simulink model "matching"  (R2015a)
settings: Solver=ode45  StartTime=0.0  StopTime=10.0  RelTol=1e-3
InitFcn:
  | %% DSPBuilder Start
  | alt_dspbuilder_update_model(bdroot)
  | %% DSPBuilder End
libraries: allblocks_alteradspbuilder2 x186
(part 1 of 2)
settings Model: Creator=ASUS  LastModifiedBy=ASUS

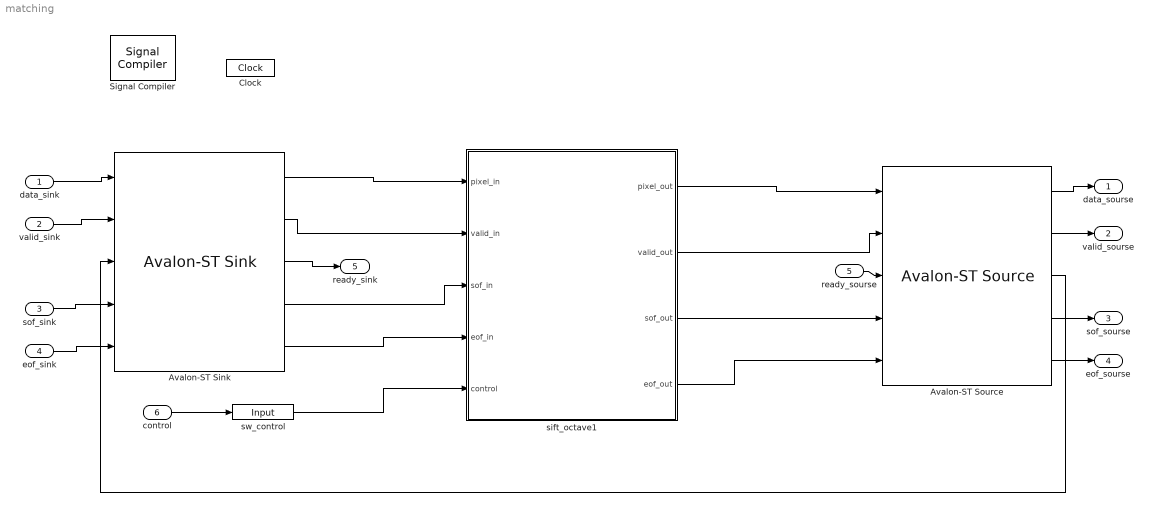
== system matching ==
  data_sink : Inport
  valid_sink : Inport  Port=2
  sof_sink : Inport  Port=3
  eof_sink : Inport  Port=4
  ready_sourse : Inport  Port=5
  control : Inport  Port=6
  Avalon-ST Sink : allblocks_alteradspbuilder2/Avalon-ST Sink  iofile=C:\Users\ASUS\Desktop\final_sift_fpga\tb_matching\matching_Avalon-ST+Sink_data.salt,C:\Users\ASUS\Desktop\final_sift_fpga\tb_matching\matching_Avalon-ST+Sink_valid.salt,C:\Users\ASUS\Desktop\final_sift_fpga\tb_matching\matching_Avalon-ST+Sink_ready.capture,C:\Users\ASUS\Desktop\final_sift_fpga\tb_matching\matching_Avalon-ST+Sink_startofpacket.salt,C:\Users\ASUS\Desktop\final_sift_fpga\tb_matching\matching_Avalon-ST+Sink_endofpacket.salt,  SpecifyClock=off  BusType=Unsigned Integer  bwl=24  bwr=0  symbolWidth=8  symbolsPerBeat=3  numOfChannels=0  numOfErrorDescriptors=0  endOfPacket=on  startOfPacket=on  empty=off  readyLatency=1  externalType=Inferred  PORTTYPE=Output
  Avalon-ST Source : allblocks_alteradspbuilder2/Avalon-ST Source  iofile=C:\Users\ASUS\Desktop\final_sift_fpga\tb_matching\matching_Avalon-ST+Source_data.capture,C:\Users\ASUS\Desktop\final_sift_fpga\tb_matching\matching_Avalon-ST+Source_valid.capture,C:\Users\ASUS\Desktop\final_sift_fpga\tb_matching\matching_Avalon-ST+Source_ready.salt,C:\Users\ASUS\Desktop\final_sift_fpga\tb_matching\matching_Avalon-ST+Source_startofpacket.capture,C:\Users\ASUS\Desktop\final_sift_fpga\tb_matching\matching_Avalon-ST+Source_endofpacket.capture,  SpecifyClock=off  BusType=Unsigned Integer  bwl=24  bwr=0  symbolWidth=8  symbolsPerBeat=3  numOfChannels=0  numOfErrorDescriptors=0  endOfPacket=on  startOfPacket=on  empty=off  readyLatency=1  externalType=Inferred  PORTTYPE=Input
  Clock : allblocks_alteradspbuilder2/Clock  ClockPeriod=10/1.5  ClockPeriodUnit=ns  SampleTime=1  ResetLatency=0  ResetRegisterCascadeDepth=0  SimulationStartCycle=5  PhaseOffset=0  Reset=aclr  ResetType=Active Low  Export=off
  Signal Compiler : allblocks_alteradspbuilder2/Signal Compiler  DeviceFamily=Cyclone IV GX  DeviceName=AUTO  DisableEarlyHDLGeneration=off  EnableSignalTap=off  SignalTapDepth=128  UseBoardBlock=off  StpUseDefaultClock=on  StpClock=Clock  ExportDir=C:\altera\16.0\quartus\dsp_builder  MAX10_ProgrammingMode=Internal Flash (SDM) Single Boot
  sift_octave1 : Subsystem
  sw_control : allblocks_alteradspbuilder2/Input  iofile=C:\Users\ASUS\Desktop\final_sift_fpga\tb_matching\matching_sw%5Fcontrol.salt  BusType=Unsigned Integer  bwl=18  bwr=0  SpecifyClock=off  PORTTYPE=Input  externalType=Inferred  allowFloatingPointOverride=on  logOutputs=off
  data_sourse : Outport
  valid_sourse : Outport  Port=2
  sof_sourse : Outport  Port=3
  eof_sourse : Outport  Port=4
  ready_sink : Outport  Port=5
  wires:
  sift_octave1/1(pixel_out) -> Avalon-ST Source/1
  Avalon-ST Sink/1 -> sift_octave1/1(pixel_in)
  Avalon-ST Sink/2 -> sift_octave1/2(valid_in)
  sift_octave1/2(valid_out) -> Avalon-ST Source/2
  sift_octave1/3(sof_out) -> Avalon-ST Source/4
  sift_octave1/4(eof_out) -> Avalon-ST Source/5
  Avalon-ST Sink/5 -> sift_octave1/4(eof_in)
  Avalon-ST Sink/4 -> sift_octave1/3(sof_in)
  Avalon-ST Source/3 -> Avalon-ST Sink/3
  Avalon-ST Source/1 -> data_sourse/1
  Avalon-ST Source/2 -> valid_sourse/1
  Avalon-ST Source/4 -> sof_sourse/1
  Avalon-ST Source/5 -> eof_sourse/1
  data_sink/1 -> Avalon-ST Sink/1
  valid_sink/1 -> Avalon-ST Sink/2
  sof_sink/1 -> Avalon-ST Sink/4
  eof_sink/1 -> Avalon-ST Sink/5
  ready_sourse/1 -> Avalon-ST Source/3
  Avalon-ST Sink/3 -> ready_sink/1
  control/1 -> sw_control/1
  sw_control/1 -> sift_octave1/5(control)

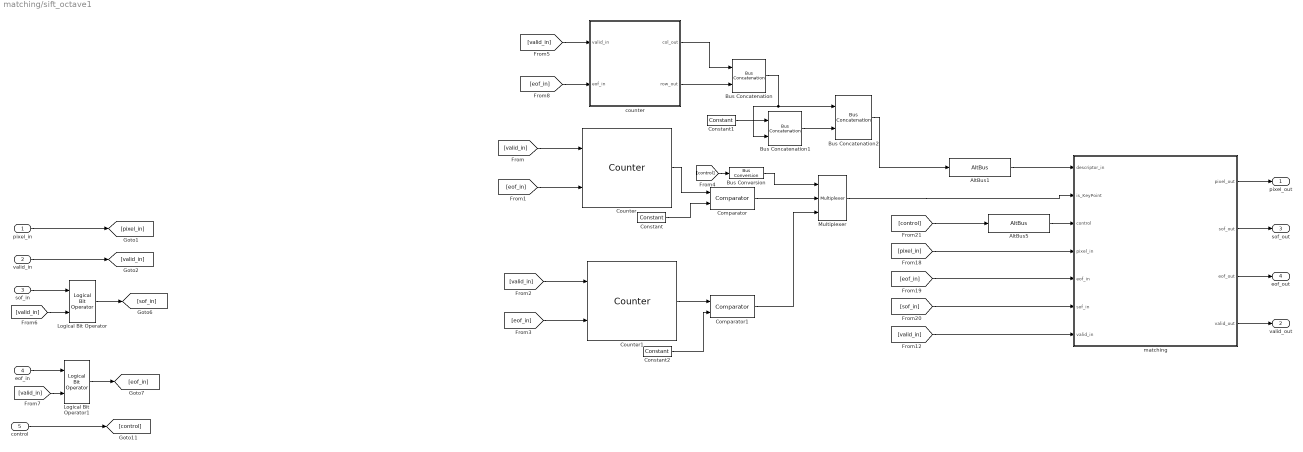
== system matching/sift_octave1 ==
  pixel_in : Inport
  valid_in : Inport  Port=2
  sof_in : Inport  Port=3
  eof_in : Inport  Port=4
  control : Inport  Port=5
  AltBus1 : allblocks_alteradspbuilder2/AltBus  BusType=Unsigned Integer  bwl=148  bwr=0  saturate=off  floatingPointInput=on  floatingPointOutput=on  logOutputs=off  logFile=C:\Users\ASUS\Desktop\final_sift_fpga\tb_matching\matching_sift%5Foctave1_AltBus1.fixedpointlog
  AltBus5 : allblocks_alteradspbuilder2/AltBus  BusType=Unsigned Integer  bwl=18  bwr=0  saturate=off  floatingPointInput=on  floatingPointOutput=on  logOutputs=off  logFile=C:\Users\ASUS\Desktop\final_sift_fpga\tb_matching\matching_sift%5Foctave1_AltBus5.fixedpointlog
  Bus Concatenation : allblocks_alteradspbuilder2/Bus Concatenation  isSigned=off  awidth=10  bwidth=10  pipeline_display=0
  Bus Concatenation1 : allblocks_alteradspbuilder2/Bus Concatenation  isSigned=off  awidth=108  bwidth=20  pipeline_display=0
  Bus Concatenation2 : allblocks_alteradspbuilder2/Bus Concatenation  isSigned=off  awidth=20  bwidth=128  pipeline_display=0
  Bus Conversion : allblocks_alteradspbuilder2/Bus Conversion  BusType=Unsigned Integer  ibwl=18  ibwr=1  bwl=1  bwr=1  bitToConnectToOutputLSB=17  round=off  saturate=off  pipeline_display=0
  Comparator : allblocks_alteradspbuilder2/Comparator  direction=a == b  pipeline_display=0  allowFloatingPointOverride=on  logOutputs=off  logFile=C:\Users\ASUS\Desktop\final_sift_fpga\tb_matching\matching_sift%5Foctave1_Comparator.fixedpointlog
  Comparator1 : allblocks_alteradspbuilder2/Comparator  direction=a == b  pipeline_display=0  allowFloatingPointOverride=on  logOutputs=off  logFile=C:\Users\ASUS\Desktop\final_sift_fpga\tb_matching\matching_sift%5Foctave1_Comparator1.fixedpointlog
  Constant : allblocks_alteradspbuilder2/Constant  mask_cst=5999  BusType=Unsigned Integer  bwl=20  bwr=0  roundMode=Truncate  satMode=Wrap  SpecifyClock=off  allowFloatingPointOverride=on  logOutputs=off  logFile=C:\Users\ASUS\Desktop\final_sift_fpga\tb_matching\matching_sift%5Foctave1_Constant.fixedpointlog
  Constant1 : allblocks_alteradspbuilder2/Constant  mask_cst=0  BusType=Unsigned Integer  bwl=108  bwr=0  roundMode=Truncate  satMode=Wrap  SpecifyClock=off  allowFloatingPointOverride=on  logOutputs=off  logFile=C:\Users\ASUS\Desktop\final_sift_fpga\tb_matching\matching_sift%5Foctave1_Constant1.fixedpointlog
  Constant2 : allblocks_alteradspbuilder2/Constant  mask_cst=4999  BusType=Unsigned Integer  bwl=20  bwr=0  roundMode=Truncate  satMode=Wrap  SpecifyClock=off  allowFloatingPointOverride=on  logOutputs=off  logFile=C:\Users\ASUS\Desktop\final_sift_fpga\tb_matching\matching_sift%5Foctave1_Constant2.fixedpointlog
  Counter : allblocks_alteradspbuilder2/Counter  BusType=Unsigned Integer  bwl=20  bwr=0  use_modulo=on  modulo=6000  SpecifyClock=off  direction=Increment  use_sload=off  use_sset=off  svalue=1  use_clk_ena=off  use_ena=on  use_sclr=on  pipeline_display=1
  Counter1 : allblocks_alteradspbuilder2/Counter  BusType=Unsigned Integer  bwl=20  bwr=0  use_modulo=on  modulo=5000  SpecifyClock=off  direction=Increment  use_sload=off  use_sset=off  svalue=1  use_clk_ena=off  use_ena=on  use_sclr=on  pipeline_display=1
  Logical Bit Operator : allblocks_alteradspbuilder2/Logical Bit Operator  LogicalOperator=AND  user_inputs=2  pipeline_display=0
  Logical Bit Operator1 : allblocks_alteradspbuilder2/Logical Bit Operator  LogicalOperator=AND  user_inputs=2  pipeline_display=0
  Multiplexer : allblocks_alteradspbuilder2/Multiplexer  numInputs=2  pipeline=0  oneHot=off  pipeline_display=0  use_ena=off  use_aclr=off  allowFloatingPointOverride=on  logOutputs=off  logFile=C:\Users\ASUS\Desktop\final_sift_fpga\tb_matching\matching_sift%5Foctave1_Multiplexer.fixedpointlog
  counter : Subsystem
  matching : Subsystem
  pixel_out : Outport
  valid_out : Outport  Port=2
  sof_out : Outport  Port=3
  eof_out : Outport  Port=4
  wires:
  control/1 -> [control]
  pixel_in/1 -> [pixel_in]
  valid_in/1 -> [valid_in]
  sof_in/1 -> Logical Bit Operator/1
  eof_in/1 -> Logical Bit Operator1/1
  AltBus1/1 -> matching/1(descriptor_in)
  [valid_in] -> matching/7(valid_in)
  [control] -> AltBus5/1
  [pixel_in] -> matching/4(pixel_in)
  [eof_in] -> matching/5(eof_in)
  [sof_in] -> matching/6(sof_in)
  AltBus5/1 -> matching/3(control)
  Comparator/1 -> Multiplexer/2
  [valid_in] -> counter/1(valid_in)
  [eof_in] -> counter/2(eof_in)
  counter/1(col_out) -> Bus Concatenation/1
  counter/2(row_out) -> Bus Concatenation/2
  Counter/1 -> Comparator/1
  [valid_in] -> Counter/1
  [eof_in] -> Counter/2
  Constant/1 -> Comparator/2
  Bus Concatenation/1 -> Bus Concatenation1/2, Bus Concatenation2/1
  Constant1/1 -> Bus Concatenation1/1
  Bus Concatenation1/1 -> Bus Concatenation2/2
  Bus Concatenation2/1 -> AltBus1/1
  Counter1/1 -> Comparator1/1
  [valid_in] -> Counter1/1
  [eof_in] -> Counter1/2
  Constant2/1 -> Comparator1/2
  Comparator1/1 -> Multiplexer/3
  Multiplexer/1 -> matching/2(is_KeyPoint)
  [control] -> Bus Conversion/1
  Bus Conversion/1 -> Multiplexer/1
  matching/1(pixel_out) -> pixel_out/1
  matching/2(sof_out) -> sof_out/1
  matching/3(eof_out) -> eof_out/1
  matching/4(valid_out) -> valid_out/1
  Logical Bit Operator/1 -> [sof_in]
  [valid_in] -> Logical Bit Operator/2
  Logical Bit Operator1/1 -> [eof_in]
  [valid_in] -> Logical Bit Operator1/2

== system matching/sift_octave1/counter ==
  valid_in : Inport
  eof_in : Inport  Port=2
  Comparator : allblocks_alteradspbuilder2/Comparator  direction=a == b  pipeline_display=0  allowFloatingPointOverride=on  logOutputs=off  logFile=C:\Users\ASUS\Desktop\PCIE_Display\custom_IP\tb_SIFT\SIFT_sift%5Foctave1_counter_Comparator.fixedpointlog
  Constant : allblocks_alteradspbuilder2/Constant  mask_cst=639  BusType=Unsigned Integer  bwl=10  bwr=0  roundMode=Truncate  satMode=Wrap  SpecifyClock=off  allowFloatingPointOverride=on  logOutputs=off  logFile=C:\Users\ASUS\Desktop\PCIE_Display\custom_IP\tb_SIFT\SIFT_sift%5Foctave1_counter_Constant.fixedpointlog
  Counter : allblocks_alteradspbuilder2/Counter  BusType=Unsigned Integer  bwl=10  bwr=0  use_modulo=on  modulo=640  SpecifyClock=off  direction=Increment  use_sload=off  use_sset=off  svalue=1  use_clk_ena=off  use_ena=on  use_sclr=on  pipeline_display=1
  Counter1 : allblocks_alteradspbuilder2/Counter  BusType=Unsigned Integer  bwl=10  bwr=0  use_modulo=on  modulo=480  SpecifyClock=off  direction=Increment  use_sload=off  use_sset=off  svalue=0  use_clk_ena=off  use_ena=on  use_sclr=on  pipeline_display=1
  Logical Bit Operator : allblocks_alteradspbuilder2/Logical Bit Operator  LogicalOperator=AND  user_inputs=2  pipeline_display=0
  col_out : Outport
  row_out : Outport  Port=2
  wires:
  [eof_in] -> Counter1/2
  Logical Bit Operator/1 -> Counter1/1
  [counter_col] -> Comparator/1
  eof_in/1 -> [eof_in]
  Constant/1 -> Comparator/2
  Comparator/1 -> Logical Bit Operator/2
  valid_in/1 -> [valid_in]
  Counter1/1 -> [counter_row]
  Counter/1 -> [counter_col]
  [valid_in] -> Logical Bit Operator/1, Counter/1
  [counter_row] -> row_out/1
  [counter_col] -> col_out/1
  [eof_in] -> Counter/2

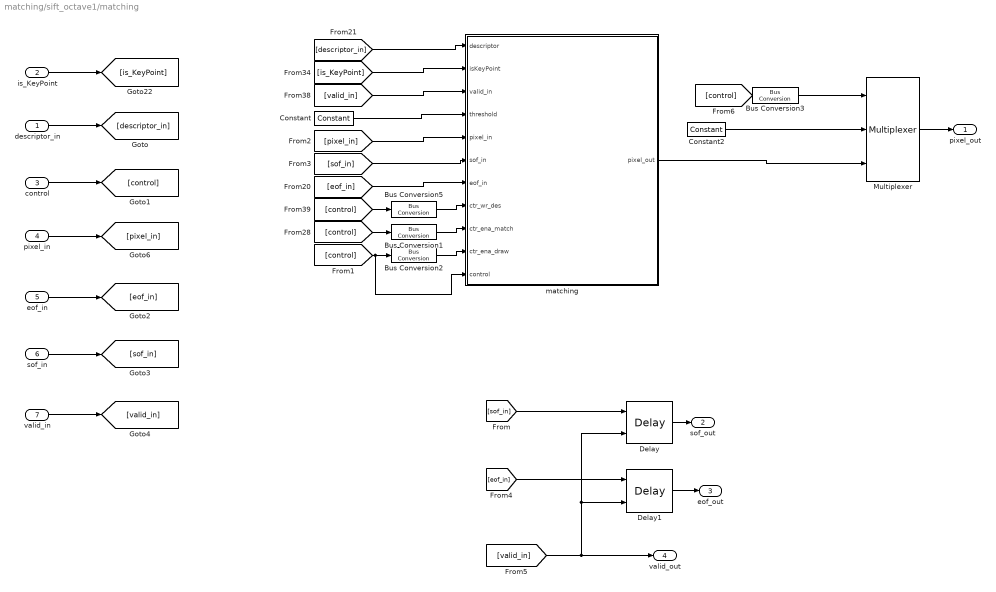
== system matching/sift_octave1/matching ==
  descriptor_in : Inport
  is_KeyPoint : Inport  Port=2
  control : Inport  Port=3
  pixel_in : Inport  Port=4
  eof_in : Inport  Port=5
  sof_in : Inport  Port=6
  valid_in : Inport  Port=7
  Bus Conversion1 : allblocks_alteradspbuilder2/Bus Conversion  BusType=Unsigned Integer  ibwl=18  ibwr=1  bwl=1  bwr=1  bitToConnectToOutputLSB=16  round=off  saturate=off  pipeline_display=0
  Bus Conversion2 : allblocks_alteradspbuilder2/Bus Conversion  BusType=Unsigned Integer  ibwl=18  ibwr=1  bwl=1  bwr=1  bitToConnectToOutputLSB=15  round=off  saturate=off  pipeline_display=0
  Bus Conversion3 : allblocks_alteradspbuilder2/Bus Conversion  BusType=Unsigned Integer  ibwl=18  ibwr=1  bwl=1  bwr=1  bitToConnectToOutputLSB=3  round=off  saturate=off  pipeline_display=0
  Bus Conversion5 : allblocks_alteradspbuilder2/Bus Conversion  BusType=Unsigned Integer  ibwl=18  ibwr=1  bwl=1  bwr=1  bitToConnectToOutputLSB=17  round=off  saturate=off  pipeline_display=0
  Constant : allblocks_alteradspbuilder2/Constant  mask_cst=1  BusType=Unsigned Integer  bwl=16  bwr=0  roundMode=Truncate  satMode=Wrap  SpecifyClock=off  allowFloatingPointOverride=on  logOutputs=off  logFile=C:\Users\ASUS\Desktop\final_sift_fpga\tb_matching\matching_sift%5Foctave1_matching_Constant.fixedpointlog
  Constant2 : allblocks_alteradspbuilder2/Constant  mask_cst=16711680  BusType=Unsigned Integer  bwl=24  bwr=0  roundMode=Truncate  satMode=Wrap  SpecifyClock=off  allowFloatingPointOverride=on  logOutputs=off  logFile=C:\Users\ASUS\Desktop\final_sift_fpga\tb_matching\matching_sift%5Foctave1_matching_Constant2.fixedpointlog
  Delay : allblocks_alteradspbuilder2/Delay  pipeline=4  pipeline_display=4  ClockPhase=1  use_ena=on  use_sclr=off  allowFloatingPointOverride=on  logOutputs=off  logFile=C:\Users\ASUS\Desktop\final_sift_fpga\tb_matching\matching_sift%5Foctave1_matching_Delay.fixedpointlog  use_init=off  reset_value=1
  Delay1 : allblocks_alteradspbuilder2/Delay  pipeline=4  pipeline_display=4  ClockPhase=1  use_ena=on  use_sclr=off  allowFloatingPointOverride=on  logOutputs=off  logFile=C:\Users\ASUS\Desktop\final_sift_fpga\tb_matching\matching_sift%5Foctave1_matching_Delay1.fixedpointlog  use_init=off  reset_value=1
  Multiplexer : allblocks_alteradspbuilder2/Multiplexer  numInputs=2  pipeline=0  oneHot=off  pipeline_display=0  use_ena=off  use_aclr=off  allowFloatingPointOverride=on  logOutputs=off  logFile=C:\Users\ASUS\Desktop\final_sift_fpga\tb_matching\matching_sift%5Foctave1_matching_Multiplexer.fixedpointlog
  matching : Subsystem
  pixel_out : Outport
  sof_out : Outport  Port=2
  eof_out : Outport  Port=3
  valid_out : Outport  Port=4
  wires:
  descriptor_in/1 -> [descriptor_in]
  control/1 -> [control]
  eof_in/1 -> [eof_in]
  sof_in/1 -> [sof_in]
  valid_in/1 -> [valid_in]
  pixel_in/1 -> [pixel_in]
  [descriptor_in] -> matching/1(descriptor)
  [is_KeyPoint] -> matching/2(isKeyPoint)
  [valid_in] -> matching/3(valid_in)
  Constant/1 -> matching/4(threshold)
  [eof_in] -> matching/7(eof_in)
  is_KeyPoint/1 -> [is_KeyPoint]
  [control] -> Bus Conversion5/1
  Bus Conversion5/1 -> matching/8(ctr_wr_des)
  [control] -> Bus Conversion1/1
  Bus Conversion1/1 -> matching/9(ctr_ena_match)
  [control] -> matching/11(control), Bus Conversion2/1
  Bus Conversion2/1 -> matching/10(ctr_ena_draw)
  [pixel_in] -> matching/5(pixel_in)
  [sof_in] -> matching/6(sof_in)
  [sof_in] -> Delay/1
  [eof_in] -> Delay1/1
  [valid_in] -> valid_out/1, Delay/2, Delay1/2
  Delay/1 -> sof_out/1
  Delay1/1 -> eof_out/1
  matching/1(pixel_out) -> Multiplexer/3
  Constant2/1 -> Multiplexer/2
  [control] -> Bus Conversion3/1
  Bus Conversion3/1 -> Multiplexer/1
  Multiplexer/1 -> pixel_out/1

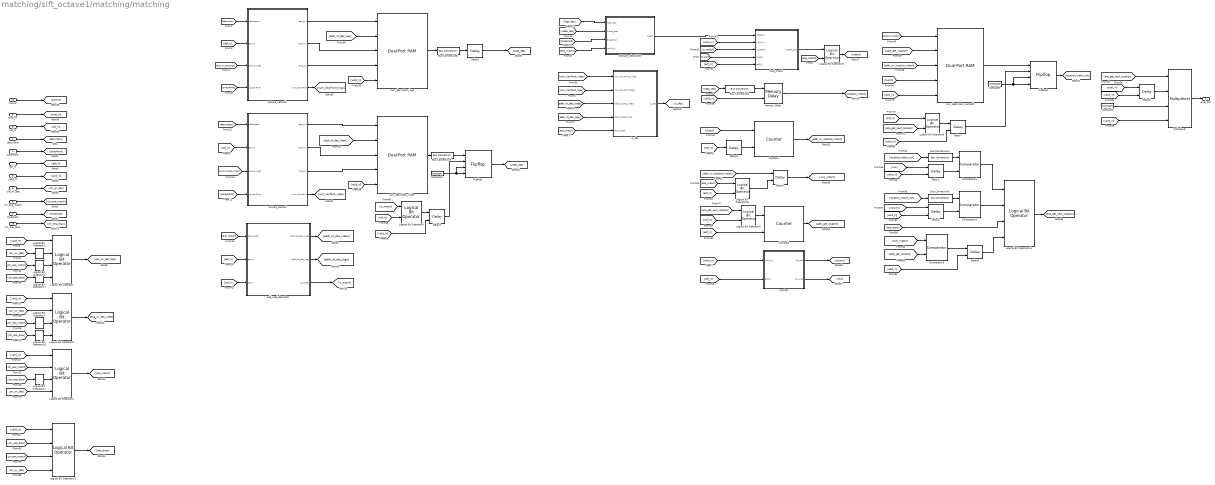
== system matching/sift_octave1/matching/matching ==
  descriptor : Inport
  isKeyPoint : Inport  Port=2
  valid_in : Inport  Port=3
  threshold : Inport  Port=4
  pixel_in : Inport  Port=5
  sof_in : Inport  Port=6
  eof_in : Inport  Port=7
  ctr_wr_des : Inport  Port=8
  ctr_ena_match : Inport  Port=9
  ctr_ena_draw : Inport  Port=10
  control : Inport  Port=11
  Bus Conversion3 : allblocks_alteradspbuilder2/Bus Conversion  BusType=Unsigned Integer  ibwl=148  ibwr=1  bwl=20  bwr=1  bitToConnectToOutputLSB=128  round=off  saturate=off  pipeline_display=0
  Bus Conversion4 : allblocks_alteradspbuilder2/Bus Conversion  BusType=Unsigned Integer  ibwl=20  ibwr=1  bwl=10  bwr=1  bitToConnectToOutputLSB=0  round=off  saturate=off  pipeline_display=0
  Bus Conversion5 : allblocks_alteradspbuilder2/Bus Conversion  BusType=Unsigned Integer  ibwl=20  ibwr=1  bwl=10  bwr=1  bitToConnectToOutputLSB=10  round=off  saturate=off  pipeline_display=0
  Bus Conversion6 : allblocks_alteradspbuilder2/Bus Conversion  BusType=Unsigned Integer  ibwl=148  ibwr=1  bwl=128  bwr=1  bitToConnectToOutputLSB=0  round=off  saturate=off  pipeline_display=0
  Bus Conversion7 : allblocks_alteradspbuilder2/Bus Conversion  BusType=Unsigned Integer  ibwl=148  ibwr=1  bwl=128  bwr=1  bitToConnectToOutputLSB=0  round=off  saturate=off  pipeline_display=0
  Comparator1 : allblocks_alteradspbuilder2/Comparator  direction=a == b  pipeline_display=0  allowFloatingPointOverride=on  logOutputs=off  logFile=C:\Users\ASUS\Desktop\final_sift_fpga\tb_matching\matching_sift%5Foctave1_matching_matching_Comparator1.fixedpointlog
  Comparator2 : allblocks_alteradspbuilder2/Comparator  direction=a == b  pipeline_display=0  allowFloatingPointOverride=on  logOutputs=off  logFile=C:\Users\ASUS\Desktop\final_sift_fpga\tb_matching\matching_sift%5Foctave1_matching_matching_Comparator2.fixedpointlog
  Comparator3 : allblocks_alteradspbuilder2/Comparator  direction=a >= b  pipeline_display=0  allowFloatingPointOverride=on  logOutputs=off  logFile=C:\Users\ASUS\Desktop\final_sift_fpga\tb_matching\matching_sift%5Foctave1_matching_matching_Comparator3.fixedpointlog
  Constant1 : allblocks_alteradspbuilder2/Constant  mask_cst=1  BusType=Single Bit  bwl=24  bwr=0  roundMode=Truncate  satMode=Wrap  SpecifyClock=off  allowFloatingPointOverride=on  logOutputs=off  logFile=C:\Users\ASUS\Desktop\final_sift_fpga\tb_matching\matching_sift%5Foctave1_matching_matching_Constant1.fixedpointlog
  Constant2 : allblocks_alteradspbuilder2/Constant  mask_cst=16711680  BusType=Unsigned Integer  bwl=24  bwr=0  roundMode=Truncate  satMode=Wrap  SpecifyClock=off  allowFloatingPointOverride=on  logOutputs=off  logFile=C:\Users\ASUS\Desktop\final_sift_fpga\tb_matching\matching_sift%5Foctave1_matching_matching_Constant2.fixedpointlog
  Constant3 : allblocks_alteradspbuilder2/Constant  mask_cst=1  BusType=Single Bit  bwl=24  bwr=0  roundMode=Truncate  satMode=Wrap  SpecifyClock=off  allowFloatingPointOverride=on  logOutputs=off  logFile=C:\Users\ASUS\Desktop\final_sift_fpga\tb_matching\matching_sift%5Foctave1_matching_matching_Constant3.fixedpointlog
  Counter1 : allblocks_alteradspbuilder2/Counter  BusType=Unsigned Integer  bwl=8  bwr=0  use_modulo=on  modulo=200  SpecifyClock=off  direction=Increment  use_sload=off  use_sset=off  svalue=1  use_clk_ena=off  use_ena=on  use_sclr=on  pipeline_display=1
  Counter2 : allblocks_alteradspbuilder2/Counter  BusType=Unsigned Integer  bwl=8  bwr=0  use_modulo=on  modulo=200  SpecifyClock=off  direction=Increment  use_sload=off  use_sset=off  svalue=1  use_clk_ena=off  use_ena=on  use_sclr=on  pipeline_display=1
  Delay1 : allblocks_alteradspbuilder2/Delay  pipeline=3  pipeline_display=3  ClockPhase=1  use_ena=on  use_sclr=off  allowFloatingPointOverride=on  logOutputs=off  logFile=C:\Users\ASUS\Desktop\final_sift_fpga\tb_matching\matching_sift%5Foctave1_matching_matching_Delay1.fixedpointlog  use_init=off  reset_value=1
  Delay2 : allblocks_alteradspbuilder2/Delay  pipeline=3  pipeline_display=3  ClockPhase=1  use_ena=on  use_sclr=off  allowFloatingPointOverride=on  logOutputs=off  logFile=C:\Users\ASUS\Desktop\final_sift_fpga\tb_matching\matching_sift%5Foctave1_matching_matching_Delay2.fixedpointlog  use_init=off  reset_value=1
  Delay3 : allblocks_alteradspbuilder2/Delay  pipeline=2  pipeline_display=2  ClockPhase=1  use_ena=on  use_sclr=off  allowFloatingPointOverride=on  logOutputs=off  logFile=C:\Users\ASUS\Desktop\final_sift_fpga\tb_matching\matching_sift%5Foctave1_matching_matching_Delay3.fixedpointlog  use_init=off  reset_value=1
  Delay4 : allblocks_alteradspbuilder2/Delay  pipeline=1  pipeline_display=1  ClockPhase=1  use_ena=on  use_sclr=off  allowFloatingPointOverride=on  logOutputs=off  logFile=C:\Users\ASUS\Desktop\final_sift_fpga\tb_matching\matching_sift%5Foctave1_matching_matching_Delay4.fixedpointlog  use_init=off  reset_value=1
  Delay5 : allblocks_alteradspbuilder2/Delay  pipeline=3  pipeline_display=3  ClockPhase=1  use_ena=on  use_sclr=off  allowFloatingPointOverride=on  logOutputs=off  logFile=C:\Users\ASUS\Desktop\final_sift_fpga\tb_matching\matching_sift%5Foctave1_matching_matching_Delay5.fixedpointlog  use_init=off  reset_value=1
  Delay6 : allblocks_alteradspbuilder2/Delay  pipeline=1  pipeline_display=1  ClockPhase=1  use_ena=off  use_sclr=off  allowFloatingPointOverride=on  logOutputs=off  logFile=C:\Users\ASUS\Desktop\final_sift_fpga\tb_matching\matching_sift%5Foctave1_matching_matching_Delay6.fixedpointlog  use_init=off  reset_value=1
  Delay7 : allblocks_alteradspbuilder2/Delay  pipeline=2  pipeline_display=2  ClockPhase=1  use_ena=on  use_sclr=off  allowFloatingPointOverride=on  logOutputs=off  logFile=C:\Users\ASUS\Desktop\final_sift_fpga\tb_matching\matching_sift%5Foctave1_matching_matching_Delay7.fixedpointlog  use_init=off  reset_value=1
  Delay8 : allblocks_alteradspbuilder2/Delay  pipeline=3  pipeline_display=3  ClockPhase=1  use_ena=on  use_sclr=off  allowFloatingPointOverride=on  logOutputs=off  logFile=C:\Users\ASUS\Desktop\final_sift_fpga\tb_matching\matching_sift%5Foctave1_matching_matching_Delay8.fixedpointlog  use_init=off  reset_value=1
  Delay9 : allblocks_alteradspbuilder2/Delay  pipeline=5  pipeline_display=5  ClockPhase=1  use_ena=off  use_sclr=off  allowFloatingPointOverride=on  logOutputs=off  logFile=C:\Users\ASUS\Desktop\final_sift_fpga\tb_matching\matching_sift%5Foctave1_matching_matching_Delay9.fixedpointlog  use_init=off  reset_value=1
  Flipflop1 : allblocks_alteradspbuilder2/Flipflop  mode=DFFE  BusType=Unsigned Integer  bwl=128  bwr=2  pipeline_display=1
  Flipflop2 : allblocks_alteradspbuilder2/Flipflop  mode=DFFE  BusType=Unsigned Integer  bwl=20  bwr=2  pipeline_display=1
  Logical Bit Operator{,2,5,14..15} (5 alike) : allblocks_alteradspbuilder2/Logical Bit Operator  LogicalOperator=AND  user_inputs=4  pipeline_display=0
  Logical Bit Operator{1,4,7,11,17..18} (6 alike) : allblocks_alteradspbuilder2/Logical Bit Operator  LogicalOperator=NOT  user_inputs=2  pipeline_display=0
  Logical Bit Operator16 : allblocks_alteradspbuilder2/Logical Bit Operator  LogicalOperator=AND  user_inputs=2  pipeline_display=0
  Logical Bit Operator3 : allblocks_alteradspbuilder2/Logical Bit Operator  LogicalOperator=OR  user_inputs=2  pipeline_display=0
  Logical Bit Operator6 : allblocks_alteradspbuilder2/Logical Bit Operator  LogicalOperator=OR  user_inputs=2  pipeline_display=0
  Logical Bit Operator8 : allblocks_alteradspbuilder2/Logical Bit Operator  LogicalOperator=OR  user_inputs=2  pipeline_display=0
  Logical Bit Operator9 : allblocks_alteradspbuilder2/Logical Bit Operator  LogicalOperator=AND  user_inputs=2  pipeline_display=0
  Memory Delay : allblocks_alteradspbuilder2/Memory Delay  BusType=Unsigned Integer  bwl=20  bwr=0  pipeline=211  pipeline_display=211  ram_type=AUTO  use_ena=on  use_sclr=off  allowFloatingPointOverride=on  logOutputs=off  logFile=C:\Users\ASUS\Desktop\final_sift_fpga\tb_matching\matching_sift%5Foctave1_matching_matching_Memory+Delay.fixedpointlog
  Multiplexer : allblocks_alteradspbuilder2/Multiplexer  numInputs=2  pipeline=1  oneHot=off  pipeline_display=1  use_ena=on  use_aclr=off  allowFloatingPointOverride=on  logOutputs=off  logFile=C:\Users\ASUS\Desktop\final_sift_fpga\tb_matching\matching_sift%5Foctave1_matching_matching_Multiplexer.fixedpointlog
  add_read_desciptor : Subsystem
  compare_descriptor : Subsystem
  counter : Subsystem
  final_match : Subsystem
  is_des : Subsystem
  picture_second : Subsystem
  picture_second1 : Subsystem
  ram_descriptor_logo : allblocks_alteradspbuilder2/Dual-Port RAM  numwords=200  BusType=Unsigned Integer  bwl=148  bwr=0  memory_type=AUTO  ram_type=DualRAM  dont_care=on  initialization=Blank  init_file=input.hex  init_array=[0:1:15]  register_outputs=on  use_ena=on  ClockPhase=1  allowFloatingPointOverride=on  logOutputs=off  logFile=C:\Users\ASUS\Desktop\final_sift_fpga\tb_matching\matching_sift%5Foctave1_matching_matching_ram%5Fdescriptor%5Flogo.fixedpointlog  pipeline_display=2
  ram_descriptor_second1 : allblocks_alteradspbuilder2/Dual-Port RAM  numwords=200  BusType=Unsigned Integer  bwl=20  bwr=0  memory_type=AUTO  ram_type=DualRAM  dont_care=on  initialization=Blank  init_file=input.hex  init_array=[0:1:15]  register_outputs=on  use_ena=on  ClockPhase=1  allowFloatingPointOverride=on  logOutputs=off  logFile=C:\Users\ASUS\Desktop\final_sift_fpga\tb_matching\matching_sift%5Foctave1_matching_matching_ram%5Fdescriptor%5Fsecond1.fixedpointlog  pipeline_display=2
  ram_descriptor_video : allblocks_alteradspbuilder2/Dual-Port RAM  numwords=1536  BusType=Unsigned Integer  bwl=148  bwr=0  memory_type=AUTO  ram_type=DualRAM  dont_care=on  initialization=Blank  init_file=input.hex  init_array=[0:1:15]  register_outputs=on  use_ena=on  ClockPhase=1  allowFloatingPointOverride=on  logOutputs=off  logFile=C:\Users\ASUS\Desktop\final_sift_fpga\tb_matching\matching_sift%5Foctave1_matching_matching_ram%5Fdescriptor%5Fvideo.fixedpointlog  pipeline_display=2
  pixel_out : Outport
  wires:
  descriptor/1 -> [descriptor]
  ctr_wr_des/1 -> [ctr_wr_des]
  eof_in/1 -> [eof_in]
  isKeyPoint/1 -> [isKeyPoint]
  valid_in/1 -> [valid_in]
  threshold/1 -> [threshold]
  Logical Bit Operator/1 -> [ena_wr_des_logo]
  [ctr_wr_des] -> Logical Bit Operator1/1
  [valid_in] -> Logical Bit Operator/1
  Logical Bit Operator1/1 -> Logical Bit Operator/2
  [ctr_ena_match] -> Logical Bit Operator4/1
  Logical Bit Operator4/1 -> Logical Bit Operator/3
  ctr_ena_match/1 -> [ctr_ena_match]
  Logical Bit Operator5/1 -> [ena_wr_des_video]
  [valid_in] -> Logical Bit Operator5/1
  [ctr_wr_des] -> Logical Bit Operator5/2
  [ctr_ena_match] -> Logical Bit Operator7/1
  Logical Bit Operator7/1 -> Logical Bit Operator5/3
  Logical Bit Operator2/1 -> [ena_match]
  [valid_in] -> Logical Bit Operator2/1
  [ctr_ena_match] -> Logical Bit Operator2/2
  ctr_ena_draw/1 -> [ctr_ena_draw]
  [ctr_ena_draw] -> Logical Bit Operator11/1
  Logical Bit Operator11/1 -> Logical Bit Operator2/3
  Logical Bit Operator15/1 -> [ena_draw]
  [valid_in] -> Logical Bit Operator15/1
  [ctr_ena_draw] -> Logical Bit Operator15/2
  pixel_in/1 -> [pixel_in]
  sof_in/1 -> [sof_in]
  [ctr_ena_draw] -> Logical Bit Operator17/1
  [ctr_ena_draw] -> Logical Bit Operator18/1
  Logical Bit Operator17/1 -> Logical Bit Operator/4
  Logical Bit Operator18/1 -> Logical Bit Operator5/4
  control/1 -> [control]
  [ctr_wr_des] -> Logical Bit Operator2/4
  [ctr_ena_match] -> Logical Bit Operator15/3
  [ctr_wr_des] -> Logical Bit Operator15/4
  [eof_in] -> picture_second/2(eof_in)
  ram_descriptor_video/1 -> Bus Conversion7/1
  [addr_rd_des_video] -> ram_descriptor_video/2
  picture_second/1(des_out) -> ram_descriptor_video/1
  picture_second/2(addr_wr) -> ram_descriptor_video/3
  [descriptor] -> picture_second/1(descriptor)
  [ena_wr_des_video] -> picture_second/3(ena_wr_des)
  [isKeyPoint] -> picture_second/4(is_KeyPoint)
  [ena_match] -> add_read_desciptor/1(ena_match)
  add_read_desciptor/1(addr_rd_des_video) -> [addr_rd_des_video]
  picture_second/3(ena_wr) -> ram_descriptor_video/4
  picture_second/4(num_KeyPoint) -> [num_KeyPoint_video]
  [eof_in] -> add_read_desciptor/2(eof_in)
  add_read_desciptor/3(is_match) -> [is_match]
  [sof_in] -> add_read_desciptor/3(sof_in)
  [descriptor] -> picture_second1/1(descriptor)
  [ena_wr_des_logo] -> picture_second1/3(ena_wr_des)
  [eof_in] -> picture_second1/2(eof_in)
  [isKeyPoint] -> picture_second1/4(is_KeyPoint)
  Multiplexer/1 -> pixel_out/1
  ram_descriptor_logo/1 -> Bus Conversion6/1
  [addr_rd_des_logo] -> ram_descriptor_logo/2
  picture_second1/1(des_out) -> ram_descriptor_logo/1
  picture_second1/2(addr_wr) -> ram_descriptor_logo/3
  picture_second1/3(ena_wr) -> ram_descriptor_logo/4
  picture_second1/4(num_KeyPoint) -> [num_KeyPoint_logo]
  add_read_desciptor/2(addr_rd_des_logo) -> [addr_rd_des_logo]
  [valid_in] -> ram_descriptor_logo/5
  [valid_in] -> ram_descriptor_video/5
  Flipflop1/1 -> [video_des]
  [is_match] -> Logical Bit Operator6/1
  [sof_in] -> Logical Bit Operator6/2
  Logical Bit Operator6/1 -> Delay3/1
  [valid_in] -> Delay3/2
  Delay3/1 -> Flipflop1/2
  Constant1/1 -> Flipflop1/3, Flipflop1/4
  Delay6/1 -> [logo_des]
  Bus Conversion6/1 -> Delay6/1
  Bus Conversion7/1 -> Flipflop1/1
  final_match/1(match_out) -> Logical Bit Operator9/1
  [pixel_in] -> Delay5/1
  [valid_in] -> Delay5/2
  Delay5/1 -> Multiplexer/2
  [valid_in] -> Multiplexer/4
  Constant2/1 -> Multiplexer/3
  [threshold] -> compare_descriptor/3(threshold)
  [ena_match] -> compare_descriptor/4(valid_in)
  [logo_des] -> compare_descriptor/1(logo_des)
  [video_des] -> compare_descriptor/2(video_des)
  compare_descriptor/1(match) -> final_match/1(match_in)
  [valid_in] -> final_match/2("valid_in ")
  [is_match] -> final_match/3(is_match)
  [is_des] -> final_match/4(is_des)
  [eof_in] -> final_match/5(eof_in)
  [num_KeyPoint_video] -> is_des/1(num_KeyPoint_video)
  [num_KeyPoint_logo] -> is_des/2(num_KeyPoint_logo)
  [addr_rd_des_video] -> is_des/3(addr_rd_des_video)
  [addr_rd_des_logo] -> is_des/4(addr_rd_des_logo)
  [ena_match] -> is_des/5(ena_match)
  is_des/1(is_des) -> [is_des]
  Bus Conversion3/1 -> Memory Delay/1
  [valid_in] -> Memory Delay/2
  [video_des] -> Bus Conversion3/1
  Counter1/1 -> [addr_wr_location_match]
  [eof_in] -> Delay9/1
  Counter2/1 -> [addr_get_location]
  [ena_get_next_location] -> Logical Bit Operator3/1
  [eof_in] -> Counter2/2
  [valid_in] -> counter/1(valid_in)
  [eof_in] -> counter/2(eof_in)
  counter/1(col_out) -> [column]
  counter/2(row_out) -> [row]
  [ena_match] -> Logical Bit Operator16/1
  [addr_wr_location_match] -> Delay4/1
  [eof_in] -> Logical Bit Operator16/2
  Logical Bit Operator16/1 -> Delay4/2
  Delay4/1 -> [num_match]
  Delay9/1 -> Counter1/2
  Logical Bit Operator3/1 -> Counter2/1
  [sof_in] -> Logical Bit Operator3/2
  Memory Delay/1 -> [location_match]
  [match] -> Counter1/1
  [ena_get_next_location] -> Multiplexer/1
  [location_match] -> ram_descriptor_second1/1
  [match] -> ram_descriptor_second1/4
  [addr_wr_location_match] -> ram_descriptor_second1/3
  ram_descriptor_second1/1 -> Flipflop2/1
  [addr_get_location] -> ram_descriptor_second1/2
  [location_match_out] -> Bus Conversion4/1
  Bus Conversion4/1 -> Comparator1/1
  [row] -> Delay1/1
  [location_match_out] -> Bus Conversion5/1
  Bus Conversion5/1 -> Comparator2/1
  Comparator2/1 -> Logical Bit Operator14/2
  Comparator1/1 -> Logical Bit Operator14/1
  [ena_draw] -> Logical Bit Operator14/3
  Logical Bit Operator14/1 -> [ena_get_next_location]
  Delay1/1 -> Comparator1/2
  [valid_in] -> Delay1/2
  [column] -> Delay2/1
  Delay2/1 -> Comparator2/2
  [valid_in] -> Delay2/2
  [num_match] -> Comparator3/1
  [addr_get_location] -> Comparator3/2
  Comparator3/1 -> Delay8/1
  [valid_in] -> ram_descriptor_second1/5
  Flipflop2/1 -> [location_match_out]
  [ena_get_next_location] -> Logical Bit Operator8/2
  [sof_in] -> Logical Bit Operator8/1
  Logical Bit Operator8/1 -> Delay7/1
  [valid_in] -> Delay7/2
  Delay7/1 -> Flipflop2/2
  Constant3/1 -> Flipflop2/3, Flipflop2/4
  Delay8/1 -> Logical Bit Operator14/4
  [valid_in] -> Delay8/2
  Logical Bit Operator9/1 -> [match]
  [ena_match] -> Logical Bit Operator9/2

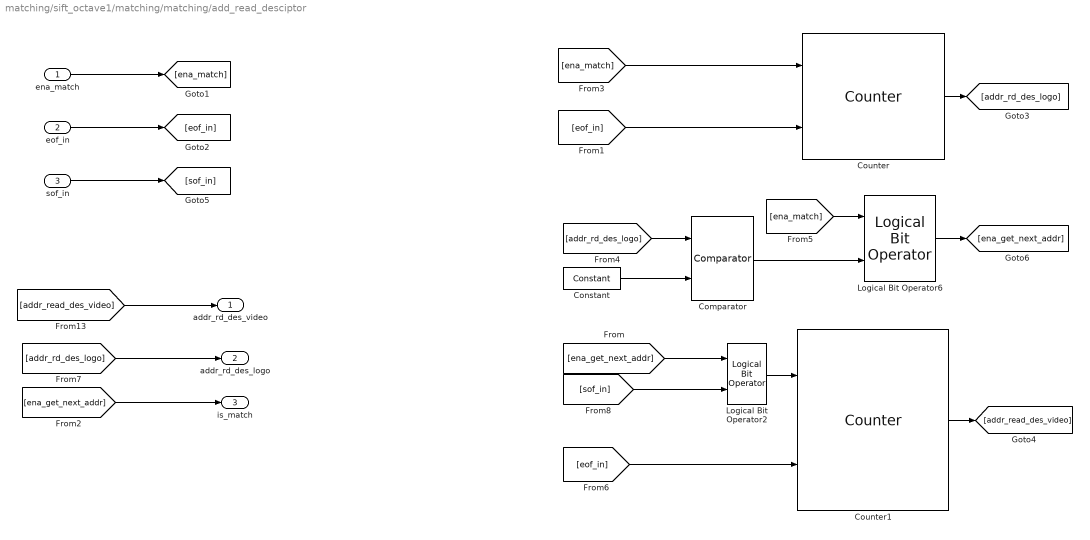
== system matching/sift_octave1/matching/matching/add_read_desciptor ==
  ena_match : Inport
  eof_in : Inport  Port=2
  sof_in : Inport  Port=3
  Comparator : allblocks_alteradspbuilder2/Comparator  direction=a == b  pipeline_display=0  allowFloatingPointOverride=on  logOutputs=off  logFile=C:\Users\ASUS\Desktop\PCIE_Display\custom_IP\tb_SIFT\SIFT_sift%5Foctave1_matching_matching_add%5Fread%5Fdesciptor_Comparator.fixedpointlog
  Constant : allblocks_alteradspbuilder2/Constant  mask_cst=199  BusType=Unsigned Integer  bwl=10  bwr=0  roundMode=Truncate  satMode=Wrap  SpecifyClock=off  allowFloatingPointOverride=on  logOutputs=off  logFile=C:\Users\ASUS\Desktop\PCIE_Display\custom_IP\tb_SIFT\SIFT_sift%5Foctave1_matching_matching_add%5Fread%5Fdesciptor_Constant.fixedpointlog
  Counter : allblocks_alteradspbuilder2/Counter  BusType=Unsigned Integer  bwl=8  bwr=0  use_modulo=on  modulo=200  SpecifyClock=off  direction=Increment  use_sload=off  use_sset=off  svalue=1  use_clk_ena=off  use_ena=on  use_sclr=on  pipeline_display=1
  Counter1 : allblocks_alteradspbuilder2/Counter  BusType=Unsigned Integer  bwl=11  bwr=0  use_modulo=on  modulo=1536  SpecifyClock=off  direction=Increment  use_sload=off  use_sset=off  svalue=0  use_clk_ena=off  use_ena=on  use_sclr=on  pipeline_display=1
  Logical Bit Operator2 : allblocks_alteradspbuilder2/Logical Bit Operator  LogicalOperator=OR  user_inputs=2  pipeline_display=0
  Logical Bit Operator6 : allblocks_alteradspbuilder2/Logical Bit Operator  LogicalOperator=AND  user_inputs=2  pipeline_display=0
  addr_rd_des_video : Outport
  addr_rd_des_logo : Outport  Port=2
  is_match : Outport  Port=3
  wires:
  [addr_rd_des_logo] -> Comparator/1
  ena_match/1 -> [ena_match]
  Constant/1 -> Comparator/2
  Counter1/1 -> [addr_read_des_video]
  Counter/1 -> [addr_rd_des_logo]
  [addr_read_des_video] -> addr_rd_des_video/1
  Comparator/1 -> Logical Bit Operator6/2
  [ena_match] -> Counter/1
  Logical Bit Operator6/1 -> [ena_get_next_addr]
  eof_in/1 -> [eof_in]
  [eof_in] -> Counter/2
  [ena_match] -> Logical Bit Operator6/1
  [ena_get_next_addr] -> is_match/1
  [eof_in] -> Counter1/2
  [ena_get_next_addr] -> Logical Bit Operator2/1
  sof_in/1 -> [sof_in]
  Logical Bit Operator2/1 -> Counter1/1
  [sof_in] -> Logical Bit Operator2/2
  [addr_rd_des_logo] -> addr_rd_des_logo/1

== system matching/sift_octave1/matching/matching/compare_descriptor ==
  logo_des : Inport
  video_des : Inport  Port=2
  threshold : Inport  Port=3
  valid_in : Inport  Port=4
  AltBus2 : allblocks_alteradspbuilder2/AltBus  BusType=Unsigned Integer  bwl=16  bwr=0  saturate=off  floatingPointInput=on  floatingPointOutput=on  logOutputs=off  logFile=C:\Users\ASUS\Desktop\final_sift_fpga\tb_matching\matching_sift%5Foctave1_matching_matching_compare%5Fdescriptor_AltBus2.fixedpointlog
  AltBus3 : allblocks_alteradspbuilder2/AltBus  BusType=Unsigned Integer  bwl=16  bwr=0  saturate=off  floatingPointInput=on  floatingPointOutput=on  logOutputs=off  logFile=C:\Users\ASUS\Desktop\final_sift_fpga\tb_matching\matching_sift%5Foctave1_matching_matching_compare%5Fdescriptor_AltBus3.fixedpointlog
  Delay : allblocks_alteradspbuilder2/Delay  pipeline=4  pipeline_display=4  ClockPhase=1  use_ena=on  use_sclr=off  allowFloatingPointOverride=on  logOutputs=off  logFile=C:\Users\ASUS\Desktop\final_sift_fpga\tb_matching\matching_sift%5Foctave1_matching_matching_compare%5Fdescriptor_Delay.fixedpointlog  use_init=off  reset_value=1
  Delay1 : allblocks_alteradspbuilder2/Delay  pipeline=1  pipeline_display=1  ClockPhase=1  use_ena=on  use_sclr=off  allowFloatingPointOverride=on  logOutputs=off  logFile=C:\Users\ASUS\Desktop\final_sift_fpga\tb_matching\matching_sift%5Foctave1_matching_matching_compare%5Fdescriptor_Delay1.fixedpointlog  use_init=off  reset_value=1
  compare : Subsystem
  get_distance : Subsystem
  match : Outport
  wires:
  [clken] -> get_distance/3(clken)
  video_des/1 -> get_distance/2(hist_in2)
  logo_des/1 -> get_distance/1(hist_in1)
  get_distance/1(distance_out) -> [distance]
  threshold/1 -> [threshold]
  Delay/1 -> AltBus3/1
  [threshold] -> AltBus2/1
  [match] -> match/1
  compare/1(match) -> Delay1/1
  AltBus2/1 -> compare/1(threshold)
  AltBus3/1 -> compare/2(distance)
  valid_in/1 -> [clken]
  [distance] -> Delay/1
  [clken] -> Delay/2
  Delay1/1 -> [match]
  [clken] -> Delay1/2

== system matching/sift_octave1/matching/matching/counter ==
  valid_in : Inport
  eof_in : Inport  Port=2
  Comparator : allblocks_alteradspbuilder2/Comparator  direction=a == b  pipeline_display=0  allowFloatingPointOverride=on  logOutputs=off  logFile=C:\Users\ASUS\Desktop\PCIE_Display\custom_IP\tb_SIFT\SIFT_sift%5Foctave1_matching_matching_counter_Comparator.fixedpointlog
  Constant : allblocks_alteradspbuilder2/Constant  mask_cst=639  BusType=Unsigned Integer  bwl=10  bwr=0  roundMode=Truncate  satMode=Wrap  SpecifyClock=off  allowFloatingPointOverride=on  logOutputs=off  logFile=C:\Users\ASUS\Desktop\PCIE_Display\custom_IP\tb_SIFT\SIFT_sift%5Foctave1_matching_matching_counter_Constant.fixedpointlog
  Counter : allblocks_alteradspbuilder2/Counter  BusType=Unsigned Integer  bwl=10  bwr=0  use_modulo=on  modulo=640  SpecifyClock=off  direction=Increment  use_sload=off  use_sset=off  svalue=1  use_clk_ena=off  use_ena=on  use_sclr=on  pipeline_display=1
  Counter1 : allblocks_alteradspbuilder2/Counter  BusType=Unsigned Integer  bwl=10  bwr=0  use_modulo=on  modulo=480  SpecifyClock=off  direction=Increment  use_sload=off  use_sset=off  svalue=0  use_clk_ena=off  use_ena=on  use_sclr=on  pipeline_display=1
  Logical Bit Operator : allblocks_alteradspbuilder2/Logical Bit Operator  LogicalOperator=AND  user_inputs=2  pipeline_display=0
  col_out : Outport
  row_out : Outport  Port=2
  wires:
  [eof_in] -> Counter1/2
  Logical Bit Operator/1 -> Counter1/1
  [counter_col] -> Comparator/1
  eof_in/1 -> [eof_in]
  Constant/1 -> Comparator/2
  Comparator/1 -> Logical Bit Operator/2
  valid_in/1 -> [valid_in]
  Counter1/1 -> [counter_row]
  Counter/1 -> [counter_col]
  [valid_in] -> Logical Bit Operator/1, Counter/1
  [counter_row] -> row_out/1
  [counter_col] -> col_out/1
  [eof_in] -> Counter/2

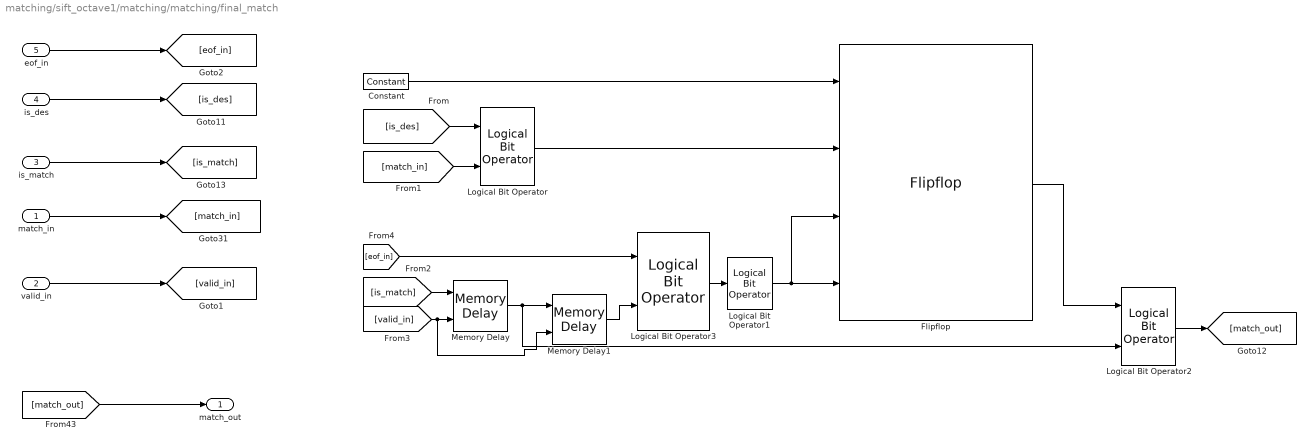
== system matching/sift_octave1/matching/matching/final_match ==
  match_in : Inport
  "valid_in " : Inport  Port=2
  is_match : Inport  Port=3
  is_des : Inport  Port=4
  eof_in : Inport  Port=5
  Constant : allblocks_alteradspbuilder2/Constant  mask_cst=1  BusType=Single Bit  bwl=8  bwr=0  roundMode=Truncate  satMode=Wrap  SpecifyClock=off  allowFloatingPointOverride=on  logOutputs=off  logFile=C:\Users\ASUS\Desktop\PCIE_Display\custom_IP\tb_SIFT\SIFT_sift%5Foctave1_matching_matching_final%5Fmatch_Constant.fixedpointlog
  Flipflop : allblocks_alteradspbuilder2/Flipflop  mode=DFFE  BusType=Single Bit  bwl=2  bwr=2  pipeline_display=1
  Logical Bit Operator : allblocks_alteradspbuilder2/Logical Bit Operator  LogicalOperator=AND  user_inputs=2  pipeline_display=0
  Logical Bit Operator1 : allblocks_alteradspbuilder2/Logical Bit Operator  LogicalOperator=NOT  user_inputs=2  pipeline_display=0
  Logical Bit Operator2 : allblocks_alteradspbuilder2/Logical Bit Operator  LogicalOperator=AND  user_inputs=2  pipeline_display=0
  Logical Bit Operator3 : allblocks_alteradspbuilder2/Logical Bit Operator  LogicalOperator=OR  user_inputs=2  pipeline_display=0
  Memory Delay : allblocks_alteradspbuilder2/Memory Delay  BusType=Unsigned Integer  bwl=1  bwr=0  pipeline=12  pipeline_display=12  ram_type=AUTO  use_ena=on  use_sclr=off  allowFloatingPointOverride=on  logOutputs=off  logFile=C:\Users\ASUS\Desktop\PCIE_Display\custom_IP\tb_SIFT\SIFT_sift%5Foctave1_matching_matching_final%5Fmatch_Memory+Delay.fixedpointlog
  Memory Delay1 : allblocks_alteradspbuilder2/Memory Delay  BusType=Unsigned Integer  bwl=1  bwr=0  pipeline=1  pipeline_display=1  ram_type=AUTO  use_ena=on  use_sclr=off  allowFloatingPointOverride=on  logOutputs=off  logFile=C:\Users\ASUS\Desktop\PCIE_Display\custom_IP\tb_SIFT\SIFT_sift%5Foctave1_matching_matching_final%5Fmatch_Memory+Delay1.fixedpointlog
  match_out : Outport
  wires:
  "valid_in "/1 -> [valid_in]
  match_in/1 -> [match_in]
  [match_out] -> match_out/1
  is_match/1 -> [is_match]
  is_des/1 -> [is_des]
  Flipflop/1 -> Logical Bit Operator2/1
  Constant/1 -> Flipflop/1
  [is_des] -> Logical Bit Operator/1
  [match_in] -> Logical Bit Operator/2
  Logical Bit Operator/1 -> Flipflop/2
  [is_match] -> Memory Delay/1
  [valid_in] -> Memory Delay1/2, Memory Delay/2
  Logical Bit Operator1/1 -> Flipflop/3, Flipflop/4
  Memory Delay/1 -> Memory Delay1/1, Logical Bit Operator2/2
  Logical Bit Operator2/1 -> [match_out]
  eof_in/1 -> [eof_in]
  Logical Bit Operator3/1 -> Logical Bit Operator1/1
  [eof_in] -> Logical Bit Operator3/1
  Memory Delay1/1 -> Logical Bit Operator3/2

== system matching/sift_octave1/matching/matching/is_des ==
  num_KeyPoint_video : Inport
  num_KeyPoint_logo : Inport  Port=2
  addr_rd_des_video : Inport  Port=3
  addr_rd_des_logo : Inport  Port=4
  ena_match : Inport  Port=5
  Comparator : allblocks_alteradspbuilder2/Comparator  direction=a >= b  pipeline_display=0  allowFloatingPointOverride=on  logOutputs=off  logFile=C:\Users\ASUS\Desktop\PCIE_Display\custom_IP\tb_SIFT\SIFT_sift%5Foctave1_matching_matching_is%5Fdes_Comparator.fixedpointlog
  Comparator6 : allblocks_alteradspbuilder2/Comparator  direction=a >= b  pipeline_display=0  allowFloatingPointOverride=on  logOutputs=off  logFile=C:\Users\ASUS\Desktop\PCIE_Display\custom_IP\tb_SIFT\SIFT_sift%5Foctave1_matching_matching_is%5Fdes_Comparator6.fixedpointlog
  Logical Bit Operator9 : allblocks_alteradspbuilder2/Logical Bit Operator  LogicalOperator=AND  user_inputs=2  pipeline_display=0
  Memory Delay1 : allblocks_alteradspbuilder2/Memory Delay  BusType=Unsigned Integer  bwl=1  bwr=0  pipeline=13  pipeline_display=13  ram_type=AUTO  use_ena=on  use_sclr=off  allowFloatingPointOverride=on  logOutputs=off  logFile=C:\Users\ASUS\Desktop\PCIE_Display\custom_IP\tb_SIFT\SIFT_sift%5Foctave1_matching_matching_is%5Fdes_Memory+Delay1.fixedpointlog
  Memory Delay2 : allblocks_alteradspbuilder2/Memory Delay  BusType=Unsigned Integer  bwl=1  bwr=0  pipeline=13  pipeline_display=13  ram_type=AUTO  use_ena=on  use_sclr=off  allowFloatingPointOverride=on  logOutputs=off  logFile=C:\Users\ASUS\Desktop\PCIE_Display\custom_IP\tb_SIFT\SIFT_sift%5Foctave1_matching_matching_is%5Fdes_Memory+Delay2.fixedpointlog
  is_des : Outport
  wires:
  [num_KeyPoint_video] -> Comparator/1
  Comparator/1 -> Memory Delay2/1
  [addr_rd_des_video] -> Comparator/2
  [ena_match] -> Memory Delay2/2
  [num_KeyPoint_logo] -> Comparator6/1
  Comparator6/1 -> Memory Delay1/1
  [addr_rd_des_logo] -> Comparator6/2
  Memory Delay2/1 -> Logical Bit Operator9/1
  Memory Delay1/1 -> Logical Bit Operator9/2
  Logical Bit Operator9/1 -> is_des/1
  [ena_match] -> Memory Delay1/2
  num_KeyPoint_video/1 -> [num_KeyPoint_video]
  num_KeyPoint_logo/1 -> [num_KeyPoint_logo]
  addr_rd_des_video/1 -> [addr_rd_des_video]
  addr_rd_des_logo/1 -> [addr_rd_des_logo]
  ena_match/1 -> [ena_match]

== system matching/sift_octave1/matching/matching/picture_second ==
  descriptor : Inport
  eof_in : Inport  Port=2
  ena_wr_des : Inport  Port=3
  is_KeyPoint : Inport  Port=4
  Constant1 : allblocks_alteradspbuilder2/Constant  mask_cst=1  BusType=Single Bit  bwl=24  bwr=0  roundMode=Truncate  satMode=Wrap  SpecifyClock=off  allowFloatingPointOverride=on  logOutputs=off  logFile=C:\Users\ASUS\Desktop\PCIE_Display\custom_IP\tb_SIFT\SIFT_sift%5Foctave1_matching_matching_picture%5Fsecond_Constant1.fixedpointlog
  Counter : allblocks_alteradspbuilder2/Counter  BusType=Unsigned Integer  bwl=11  bwr=0  use_modulo=on  modulo=1536  SpecifyClock=off  direction=Increment  use_sload=off  use_sset=off  svalue=1  use_clk_ena=off  use_ena=on  use_sclr=on  pipeline_display=1
  Delay1 : allblocks_alteradspbuilder2/Delay  pipeline=1  pipeline_display=1  ClockPhase=1  use_ena=on  use_sclr=off  allowFloatingPointOverride=on  logOutputs=off  logFile=C:\Users\ASUS\Desktop\PCIE_Display\custom_IP\tb_SIFT\SIFT_sift%5Foctave1_matching_matching_picture%5Fsecond_Delay1.fixedpointlog  use_init=off  reset_value=1
  Delay2 : allblocks_alteradspbuilder2/Delay  pipeline=5  pipeline_display=5  ClockPhase=1  use_ena=on  use_sclr=off  allowFloatingPointOverride=on  logOutputs=off  logFile=C:\Users\ASUS\Desktop\PCIE_Display\custom_IP\tb_SIFT\SIFT_sift%5Foctave1_matching_matching_picture%5Fsecond_Delay2.fixedpointlog  use_init=off  reset_value=1
  Delay3 : allblocks_alteradspbuilder2/Delay  pipeline=1  pipeline_display=1  ClockPhase=1  use_ena=on  use_sclr=off  allowFloatingPointOverride=on  logOutputs=off  logFile=C:\Users\ASUS\Desktop\PCIE_Display\custom_IP\tb_SIFT\SIFT_sift%5Foctave1_matching_matching_picture%5Fsecond_Delay3.fixedpointlog  use_init=off  reset_value=1
  Delay4 : allblocks_alteradspbuilder2/Delay  pipeline=1  pipeline_display=1  ClockPhase=1  use_ena=on  use_sclr=off  allowFloatingPointOverride=on  logOutputs=off  logFile=C:\Users\ASUS\Desktop\PCIE_Display\custom_IP\tb_SIFT\SIFT_sift%5Foctave1_matching_matching_picture%5Fsecond_Delay4.fixedpointlog  use_init=off  reset_value=1
  Flipflop : allblocks_alteradspbuilder2/Flipflop  mode=DFFE  BusType=Unsigned Integer  bwl=148  bwr=2  pipeline_display=1
  Logical Bit Operator1 : allblocks_alteradspbuilder2/Logical Bit Operator  LogicalOperator=AND  user_inputs=2  pipeline_display=0
  Logical Bit Operator4 : allblocks_alteradspbuilder2/Logical Bit Operator  LogicalOperator=AND  user_inputs=2  pipeline_display=0
  des_out : Outport
  addr_wr : Outport  Port=2
  ena_wr : Outport  Port=3
  num_KeyPoint : Outport  Port=4
  wires:
  descriptor/1 -> Flipflop/1
  Logical Bit Operator4/1 -> Flipflop/2, Delay3/1, Counter/1
  is_KeyPoint/1 -> Logical Bit Operator4/1
  Delay1/1 -> num_KeyPoint/1
  Counter/1 -> Delay4/1, Delay1/1
  Delay2/1 -> Counter/2
  eof_in/1 -> Logical Bit Operator1/1, Delay2/1
  ena_wr_des/1 -> Logical Bit Operator1/2, Delay2/2, Logical Bit Operator4/2, Delay4/2, Delay3/2
  Logical Bit Operator1/1 -> Delay1/2
  Flipflop/1 -> des_out/1
  Constant1/1 -> Flipflop/3, Flipflop/4
  Delay3/1 -> ena_wr/1
  Delay4/1 -> addr_wr/1

== system matching/sift_octave1/matching/matching/picture_second1 ==
  descriptor : Inport
  eof_in : Inport  Port=2
  ena_wr_des : Inport  Port=3
  is_KeyPoint : Inport  Port=4
  Constant1 : allblocks_alteradspbuilder2/Constant  mask_cst=1  BusType=Single Bit  bwl=24  bwr=0  roundMode=Truncate  satMode=Wrap  SpecifyClock=off  allowFloatingPointOverride=on  logOutputs=off  logFile=C:\Users\ASUS\Desktop\PCIE_Display\custom_IP\tb_SIFT\SIFT_sift%5Foctave1_matching_matching_picture%5Fsecond1_Constant1.fixedpointlog
  Counter : allblocks_alteradspbuilder2/Counter  BusType=Unsigned Integer  bwl=8  bwr=0  use_modulo=on  modulo=200  SpecifyClock=off  direction=Increment  use_sload=off  use_sset=off  svalue=1  use_clk_ena=off  use_ena=on  use_sclr=on  pipeline_display=1
  Delay1 : allblocks_alteradspbuilder2/Delay  pipeline=1  pipeline_display=1  ClockPhase=1  use_ena=on  use_sclr=off  allowFloatingPointOverride=on  logOutputs=off  logFile=C:\Users\ASUS\Desktop\PCIE_Display\custom_IP\tb_SIFT\SIFT_sift%5Foctave1_matching_matching_picture%5Fsecond1_Delay1.fixedpointlog  use_init=off  reset_value=1
  Delay2 : allblocks_alteradspbuilder2/Delay  pipeline=5  pipeline_display=5  ClockPhase=1  use_ena=on  use_sclr=off  allowFloatingPointOverride=on  logOutputs=off  logFile=C:\Users\ASUS\Desktop\PCIE_Display\custom_IP\tb_SIFT\SIFT_sift%5Foctave1_matching_matching_picture%5Fsecond1_Delay2.fixedpointlog  use_init=off  reset_value=1
  Delay3 : allblocks_alteradspbuilder2/Delay  pipeline=1  pipeline_display=1  ClockPhase=1  use_ena=on  use_sclr=off  allowFloatingPointOverride=on  logOutputs=off  logFile=C:\Users\ASUS\Desktop\PCIE_Display\custom_IP\tb_SIFT\SIFT_sift%5Foctave1_matching_matching_picture%5Fsecond1_Delay3.fixedpointlog  use_init=off  reset_value=1
  Delay4 : allblocks_alteradspbuilder2/Delay  pipeline=1  pipeline_display=1  ClockPhase=1  use_ena=on  use_sclr=off  allowFloatingPointOverride=on  logOutputs=off  logFile=C:\Users\ASUS\Desktop\PCIE_Display\custom_IP\tb_SIFT\SIFT_sift%5Foctave1_matching_matching_picture%5Fsecond1_Delay4.fixedpointlog  use_init=off  reset_value=1
  Flipflop : allblocks_alteradspbuilder2/Flipflop  mode=DFFE  BusType=Unsigned Integer  bwl=148  bwr=2  pipeline_display=1
  Logical Bit Operator1 : allblocks_alteradspbuilder2/Logical Bit Operator  LogicalOperator=AND  user_inputs=2  pipeline_display=0
  Logical Bit Operator4 : allblocks_alteradspbuilder2/Logical Bit Operator  LogicalOperator=AND  user_inputs=2  pipeline_display=0
  des_out : Outport
  addr_wr : Outport  Port=2
  ena_wr : Outport  Port=3
  num_KeyPoint : Outport  Port=4
  wires:
  descriptor/1 -> Flipflop/1
  Logical Bit Operator4/1 -> Flipflop/2, Delay3/1, Counter/1
  is_KeyPoint/1 -> Logical Bit Operator4/1
  Delay1/1 -> num_KeyPoint/1
  Counter/1 -> Delay4/1, Delay1/1
  Delay2/1 -> Counter/2
  eof_in/1 -> Logical Bit Operator1/1, Delay2/1
  ena_wr_des/1 -> Logical Bit Operator1/2, Delay2/2, Logical Bit Operator4/2, Delay4/2, Delay3/2
  Logical Bit Operator1/1 -> Delay1/2
  Flipflop/1 -> des_out/1
  Constant1/1 -> Flipflop/3, Flipflop/4
  Delay3/1 -> ena_wr/1
  Delay4/1 -> addr_wr/1

== system matching/sift_octave1/matching/matching/compare_descriptor/compare ==
  threshold : Inport
  distance : Inport  Port=2
  Comparator : allblocks_alteradspbuilder2/Comparator  direction=a > b  pipeline_display=0  allowFloatingPointOverride=on  logOutputs=off  logFile=C:\Users\ASUS\Desktop\final_sift_fpga\tb_matching\matching_sift%5Foctave1_matching_matching_compare%5Fdescriptor_compare_Comparator.fixedpointlog
  match : Outport
  wires:
  threshold/1 -> [threshold]
  distance/1 -> [distance]
  [match] -> match/1
  [threshold] -> Comparator/1
  [distance] -> Comparator/2
  Comparator/1 -> [match]
